simulink model "ZRD_laengs_Simulator_einfach"  (R2021a)
settings: Solver=VariableStepAuto  StartTime=0.0  StopTime=10.0  RelTol=1e-3
values from neighbouring files (symbols this model uses):
  a0 = 0    [ZRD_laengs.m]    (also in ZRD_laengsbewegung.m = 0.0062)
  g = 9.81    [ZRD_laengs.m]    (also in ZRD_laengsbewegung.m; ZRD_seitenbewegung.m)
  i_f = 0    [ZRD_laengs.m]    (also in ZRD_laengsbewegung.m)
  Ma = -0.3215    [ZRD_laengs.m]    (also in ZRD_laengsbewegung.m = xhat(8))
  Mdf = -1.9727    [ZRD_laengs.m]    (also in ZRD_laengsbewegung.m = xhat(12))
  Meta = -0.0967    [ZRD_laengs.m]    (also in ZRD_laengsbewegung.m = xhat(11))
  Mq = 3.3984    [ZRD_laengs.m]    (also in ZRD_laengsbewegung.m = xhat(9))
  Mv = 5.2744    [ZRD_laengs.m]    (also in ZRD_laengsbewegung.m = xhat(10))
  V0 = 26.9962    [ZRD_laengs.m]    (also in ZRD_laengsbewegung.m = 26.9978; ZRD_seitenbewegung.m = 30)
  x0 = [a0 0 V0 0]    [ZRD_laengs.m]    (also in ZRD_laengsbewegung.m = [x1filt(1);x2filt(1);x3filt(1);x4filt(1)])
  Xa = -3.6481    [ZRD_laengs.m]    (also in ZRD_laengsbewegung.m = xhat(1))
  Xdf = 2.8712    [ZRD_laengs.m]    (also in ZRD_laengsbewegung.m = xhat(4))
  Xeta = -0.5580    (= -0.558)    [ZRD_laengs.m]    (also in ZRD_laengsbewegung.m = xhat(3))
  Xv = 6.7118    [ZRD_laengs.m]    (also in ZRD_laengsbewegung.m = xhat(2))
  Za = 9.9196    [ZRD_laengs.m]    (also in ZRD_laengsbewegung.m = xhat(5))
  Zeta = 0.8461    [ZRD_laengs.m]    (also in ZRD_laengsbewegung.m = xhat(7))
  Zv = -6.3420    (= -6.342)    [ZRD_laengs.m]    (also in ZRD_laengsbewegung.m = xhat(6))
settings Model: Creator=Florian  LastModifiedBy=Fabrizio
settings SolverCC: AlgebraicLoopSolver=TrustRegion
settings DebuggingCC: SFMachineParentedDataDiag=warning

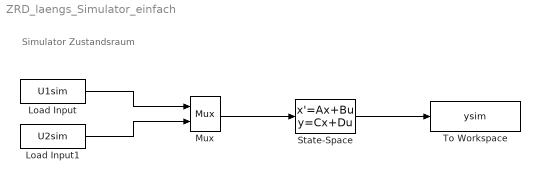
== system ZRD_laengs_Simulator_einfach ==
  note: Simulator Zustandsraum
  Load Input : FromWorkspace  VariableName=U1sim  SampleTime=-1
  Load Input1 : FromWorkspace  VariableName=U2sim  SampleTime=-1
  Mux : Mux  Inputs=2
  State-Space : StateSpace  A=[Za/V0, 1, Zv/V0, 0; Ma, Mq, Mv, 0; Xa, 0, Xv, -g; -Za/V0, 0, -Zv/V0, 0]  B=[Zeta/V0, -Xdf/V0*sin(a0+i_f); Meta, Mdf; Xeta, Xdf*cos(a0+i_f); -Zeta/V0, Xdf/V0*sin(a0+i_f)]  C=eye(4,4);  D=zeros(4,2)  InitialCondition=x0
  To Workspace : ToWorkspace  VariableName=ysim  SampleTime=-1
  wires:
  Mux/1 -> State-Space/1
  State-Space/1 -> To Workspace/1
  Load Input/1 -> Mux/1
  Load Input1/1 -> Mux/2
